simulink model "FCS_lab_1_exx1"  (R2018a)
settings: Solver=ode45  StartTime=0.0  StopTime=10  RelTol=1e-3
settings Model: Creator=Muhammad Hamza Zia  LastModifiedBy=Muhammad Hamza Zia

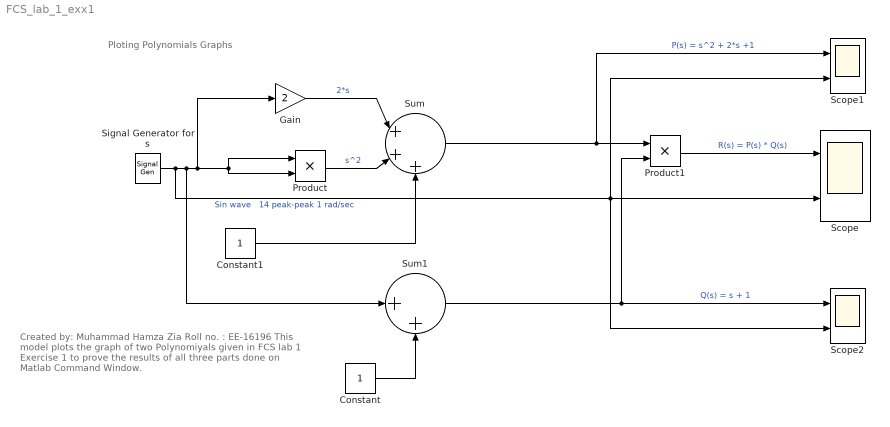
== system FCS_lab_1_exx1 ==
  note: Created by: Muhammad Hamza Zia
      | Roll no. : EE-16196
      |
      | This model plots the graph of two Polynomiyals given in
      | FCS lab 1 Exercise 1 to prove the results of all three parts
      | done on Matlab Command Window.
  note: Ploting Polynomials Graphs
  Constant : Constant
  Constant1 : Constant
  Gain : Gain  Gain=2  RndMeth=Round
  Product : Product  RndMeth=Round
  Product1 : Product  RndMeth=Round
  Scope : Scope  NumInputPorts=2
  Scope1 : Scope  NumInputPorts=2
  Scope2 : Scope  NumInputPorts=2
  Signal Generator for s : SignalGenerator  Amplitude=7  Units=rad/sec
  Sum : Sum  Inputs=|+++  RndMeth=Round
  Sum1 : Sum  Inputs=|++  RndMeth=Round
  wires:
  Signal Generator for s/1 -> Scope/2, Scope2/2, Scope1/2, Sum1/1, Gain/1, Product/2, Product/1  "Sin wave   14 peak-peak 1 rad/sec"
  Constant1/1 -> Sum/3
  Product/1 -> Sum/2  "s^2"
  Gain/1 -> Sum/1  "2*s"
  Product1/1 -> Scope/1  "R(s) = P(s) * Q(s)"
  Sum1/1 -> Product1/2, Scope2/1  "Q(s) = s + 1"
  Sum/1 -> Product1/1, Scope1/1  "P(s) = s^2 + 2*s +1"
  Constant/1 -> Sum1/2
